simulink model "motor_modeling"  (R2023a)
settings: Solver=VariableStepAuto  StartTime=0.0  StopTime=10.0  RelTol=1e-3
values from neighbouring files (symbols this model uses):
  b = 0.1    [homeworkone.m]    (also in robotics_0911.m)
  J = 0.2    [homeworkone.m]    (also in robotics_0911.m)
  Ke = 1    [homeworkone.m]    (also in robotics_0911.m)
  Kt = 1    [homeworkone.m]    (also in robotics_0911.m)
  La = 1    [homeworkone.m]    (also in robotics_0911.m)
  Ra = 0.01    [homeworkone.m]    (also in robotics_0911.m)
  Tl = 0    [homeworkone.m]    (also in robotics_0911.m)
  Va = 1    [homeworkone.m]    (also in robotics_0911.m)
settings Model: Creator=junseo  LastModifiedBy=junseo

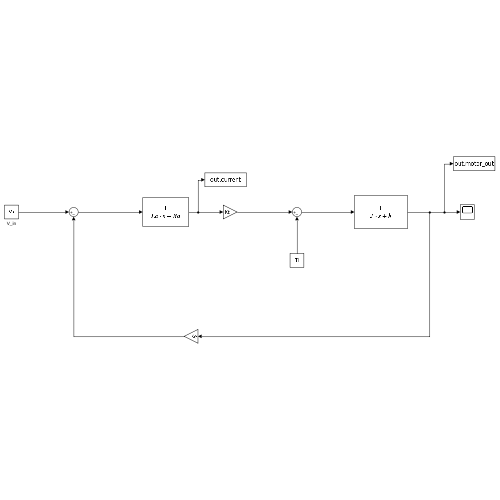
[thumbnail: Simulink's stored preview of the top-level diagram]
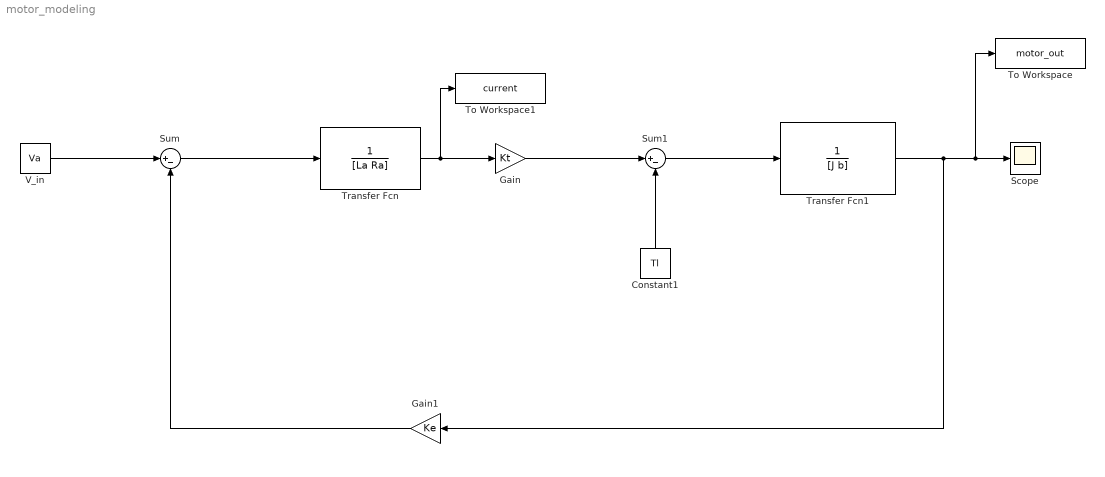
== system motor_modeling ==
  Constant1 : Constant  Value=Tl
  Gain : Gain  Gain=Kt
  Gain1 : Gain  Gain=Ke
  Scope : Scope
  Sum : Sum  Inputs=|+-
  Sum1 : Sum  Inputs=|+-
  To Workspace : ToWorkspace  VariableName=motor_out  SaveFormat=Timeseries  SampleTime=-1
  To Workspace1 : ToWorkspace  VariableName=current  SaveFormat=Timeseries  SampleTime=-1
  Transfer Fcn : TransferFcn  Denominator=[La Ra]
  Transfer Fcn1 : TransferFcn  Denominator=[J b]
  V_in : Constant  Value=Va
  wires:
  V_in/1 -> Sum/1
  Sum/1 -> Transfer Fcn/1
  Transfer Fcn/1 -> To Workspace1/1, Gain/1
  Gain/1 -> Sum1/1
  Constant1/1 -> Sum1/2
  Sum1/1 -> Transfer Fcn1/1
  Transfer Fcn1/1 -> Gain1/1, To Workspace/1, Scope/1
  Gain1/1 -> Sum/2
